simulink model "RIP"  (R2023b)
settings: Solver=ode23t  StartTime=0.0  StopTime=inf  RelTol=1e-3
model workspace: external: MATLAB File D:\AHMED\ASU\STUDENT\5. SENIOR 2\Semester 9\Hybrid Systems Control\Major Task\5. Simulink & GUI (V2)\Simulation\RIP_DataFile.m (data not in the file)
undefined symbols (not defined in the file or in its folder): k, smiData, X, Y, Z
libraries: sm_lib x16, nesl_utility x7, ee_lib x5, fl_lib x4, eeGeneralControl x2
settings Model: Creator=ahmed  LastModifiedBy=ahmed
settings ExplorerConfigSet: InternalSimMechanicsExplorerSettings="<ExplorerConfiguration><canonicalview>planar_xy</canonicalview><AnimationSetting><BasePlaybackSpeed>1.0</BasePlaybackSpeed><PlaybackSpeedFactor>1.0</PlaybackSpeedFactor></AnimationSetting><TilePanel><TileInfo><Tiles Columns=\"1\" Count=\"1\" Rows=\"1\"><Column Weight=\"1\"/><Row Weight=\"1\"/><Tile Height=\"1\" Width=\"1\" X=\"0\" Y=\"0\"/></Tiles></TileInfo><SceneInfo><SceneViewer><BGColor><R>0.60000002384185791</R><G>0.60000002384185791</G><B>0.60000002384185791</B></BGColor><Camera><DoPerspective>off</DoPerspective><Position><X>0.452835062728077831</X><Y>0.750380680384863274</Y><Z>0.622835063996346916</Z></Position><Center><X>-0.124515206461548039</X><Y>0.173030411195237543</Y><Z>0.0454847948067210878</Z></Center><Up><X>-0.408248290463863073</X><Y>0.816496580927726145</Y><Z>-0.408248290463863073</Z></Up><ViewLimDist>1</ViewLimDist><YLim>0.255279300212860105</YLim><XLim>0.46883025327554112</XLim></Camera></SceneViewer></SceneInfo></TilePanel><MechEditorPanel><Cameras/><GfxPanelCameraMap/><VideoCreator><PlaybackSpeedRatio>1.0</PlaybackSpeedRatio><FrameRate>30</FrameRate><VideoFormat>Motion JPEG AVI</VideoFormat><FrameSize>auto</FrameSize></VideoCreator></MechEditorPanel></ExplorerConfiguration>"

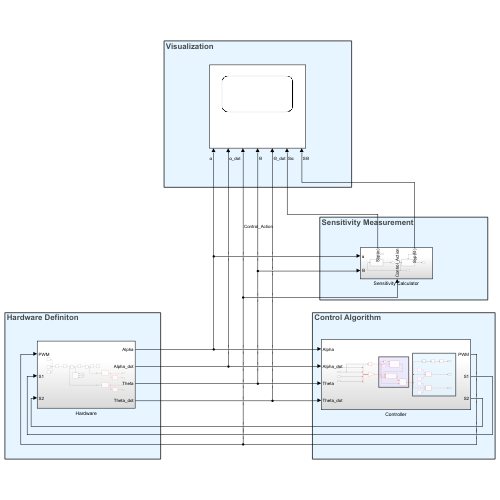
[thumbnail: Simulink's stored preview of the top-level diagram]
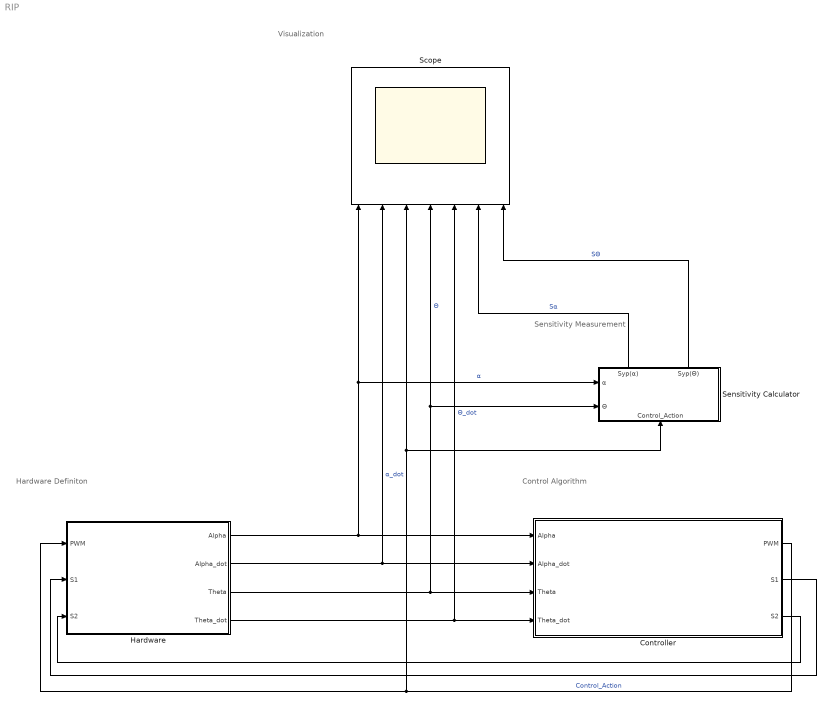
== system RIP ==
  note: Visualization
  note: Control Algorithm
  note: Hardware Definiton
  note: Sensitivity Measurement
  Controller : Subsystem
  Hardware : Subsystem
  Scope : Scope  NumInputPorts=7
  Sensitivity Calculator : Subsystem
      settings: PortSchema="{\"entries\":[{\"content\":{\"sides\":[{\"content\":{\"connectorIds\":[\"In1\",\"In2\"]},\"type\":\"ConnectorPlacement.EquallySpacedRectSide\",\"uuid\":\"a2b76d68-7d10-4964-b793-c2b104dfa3db\"},{\"content\":{\"side\":\"RIGHT\"},\"type\":\"ConnectorPlacement.EquallySpacedRectSide\",\"uuid\":\"40182234-6568-4180-b40e-3a35cefd8a8d\"},{\"content\":{\"connectorIds\":[\"Out1\",\"Out2\"],\"side\":\"TOP\"},\"type\":\"ConnectorPlacement.EquallySpacedRectSide\",\"uuid\":\"a20c4198-3069-423f-ae66-29ef70cd25fc\"},{\"content\":{\"connectorIds\":[\"In3\"],\"side\":\"BOTTOM\"},\"type\":\"ConnectorPlacement.EquallySpacedRectSide\",\"uuid\":\"777a26e0-898e-40e7-afe2-be20485a2fc9\"}]},\"type\":\"ConnectorPlacement.EquallySpacedConnector\",\"uuid\":\"2eeb0501-ac65-4270-abcc-9f050e1f1400\"}],\"packageUris\":[\"http://schema.mathworks.com/mf0/Connector/R2020b\"],\"version\":\"1.0\"}"
  wires:
  Hardware/1(Alpha) -> Controller/1(Alpha), Scope/1, Sensitivity Calculator/1(α)  "α"
  Hardware/2(Alpha_dot) -> Controller/2(Alpha_dot), Scope/2  "α_dot"
  Hardware/3(Theta) -> Controller/3(Theta), Sensitivity Calculator/2(Θ), Scope/4  "Θ"
  Hardware/4(Theta_dot) -> Controller/4(Theta_dot), Scope/5  "Θ_dot"
  Controller/1(PWM) -> Scope/3, Sensitivity Calculator/3(Control_Action), Hardware/1(PWM)  "Control_Action"
  Controller/2(S1) -> Hardware/2(S1)
  Controller/3(S2) -> Hardware/3(S2)
  Sensitivity Calculator/1(Syp(α)) -> Scope/6  "Sα"
  Sensitivity Calculator/2(Syp(Θ)) -> Scope/7  "SΘ"

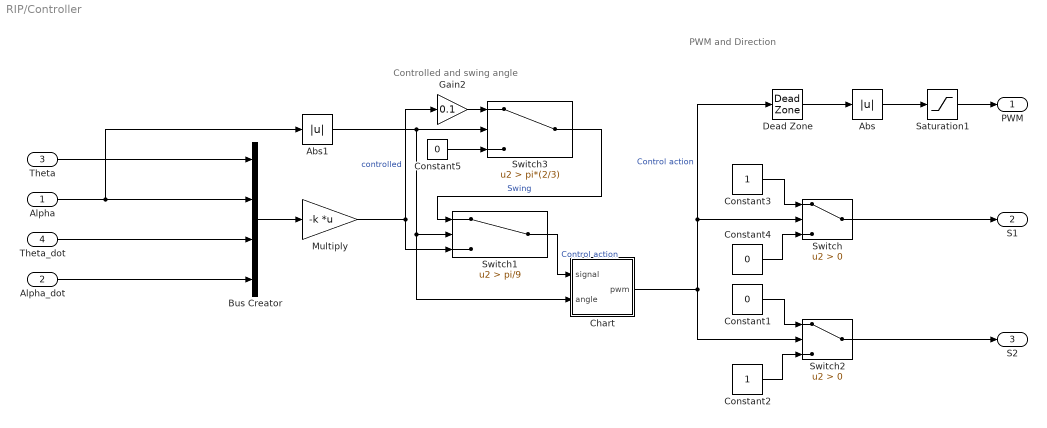
== system RIP/Controller ==
  note: Controlled and swing angle
  note: PWM and Direction
  Alpha : Inport
  Alpha_dot : Inport  Port=2
  Theta : Inport  Port=3
  Theta_dot : Inport  Port=4
  Abs : Abs  OutDataTypeStr=double  SaturateOnIntegerOverflow=off
  Abs1 : Abs  OutDataTypeStr=double  SaturateOnIntegerOverflow=off
  Bus Creator : BusCreator  Inputs=4
  Chart : Stateflow chart  TreatAsAtomicUnit=on  SystemSampleTime=0.001
      settings: PortSchema="{\"entries\":[{\"content\":{\"sides\":[{\"content\":{\"connectorIds\":[\"In2\",\"In1\"]},\"type\":\"ConnectorPlacement.EquallySpacedRectSide\",\"uuid\":\"28e2c2a8-bb0f-48a1-9e94-8475c8c1f5fa\"},{\"content\":{\"connectorIds\":[\"Out1\"],\"side\":\"RIGHT\"},\"type\":\"ConnectorPlacement.EquallySpacedRectSide\",\"uuid\":\"685929b8-ebaf-43fb-a3f1-f9f50dd919ab\"},{\"content\":{\"side\":\"TOP\"},\"type\":\"ConnectorPlacement.EquallySpacedRectSide\",\"uuid\":\"2e9fc888-3b47-4e34-86c2-38ebf694bde1\"}]},\"type\":\"ConnectorPlacement.EquallySpacedConnector\",\"uuid\":\"7dd89bc6-9eab-4521-81b3-1baa801bda82\"}],\"packageUris\":[\"http://schema.mathworks.com/mf0/Connector/R2020b\"],\"version\":\"1.0\"}"
  Constant1 : Constant  Value=0
  Constant2 : Constant
  Constant3 : Constant
  Constant4 : Constant  Value=0
  Constant5 : Constant  Value=0
  Dead Zone : DeadZone  LowerValue=-0  UpperValue=0
  Gain2 : Gain  Gain=0.1  OutDataTypeStr=double
  Multiply : Gain  Gain=-k  Multiplication=Matrix(K*u) (u vector)  OutDataTypeStr=double
  Saturation1 : Saturate  UpperLimit=255  LowerLimit=0
  Switch : Switch  Criteria=u2 > Threshold  OutDataTypeStr=double  SaturateOnIntegerOverflow=off  InputSameDT=off
  Switch1 : Switch  Criteria=u2 > Threshold  Threshold=pi/9  OutDataTypeStr=double  SaturateOnIntegerOverflow=off  InputSameDT=off
  Switch2 : Switch  Criteria=u2 > Threshold  OutDataTypeStr=double  SaturateOnIntegerOverflow=off  InputSameDT=off
  Switch3 : Switch  Criteria=u2 > Threshold  Threshold=pi*(2/3)  OutDataTypeStr=double  SaturateOnIntegerOverflow=off  InputSameDT=off
  PWM : Outport
  S1 : Outport  Port=2
  S2 : Outport  Port=3
  wires:
  Switch3/1 -> Switch1/1  "Swing"
  Bus Creator/1 -> Multiply/1
  Constant5/1 -> Switch3/3
  Abs1/1 -> Chart/1(angle), Switch1/2, Switch3/2
  Switch1/1 -> Chart/2(signal)  "Control action"
  Abs/1 -> Saturation1/1
  Constant4/1 -> Switch/3
  Multiply/1 -> Switch1/3, Gain2/1  "controlled"
  Chart/1(pwm) -> Switch2/2, Dead Zone/1, Switch/2  "Control action"
  Constant3/1 -> Switch/1
  Gain2/1 -> Switch3/1
  Theta_dot/1 -> Bus Creator/3
  Alpha/1 -> Abs1/1, Bus Creator/2
  Alpha_dot/1 -> Bus Creator/4
  Theta/1 -> Bus Creator/1
  Constant2/1 -> Switch2/3
  Constant1/1 -> Switch2/1
  Switch/1 -> S1/1
  Switch2/1 -> S2/1
  Saturation1/1 -> PWM/1
  Dead Zone/1 -> Abs/1

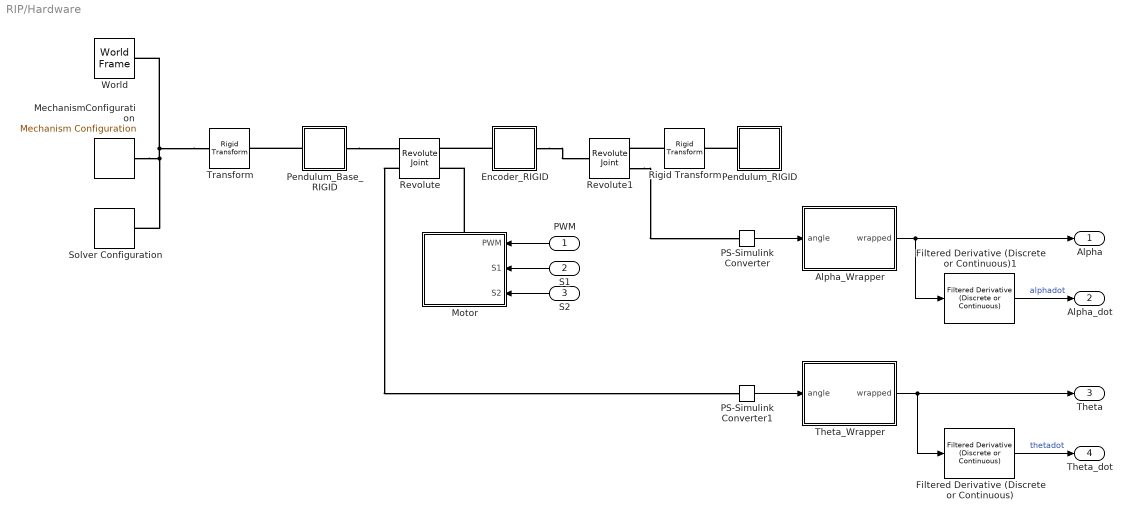
== system RIP/Hardware ==
  PWM : Inport
  S1 : Inport  Port=2
  S2 : Inport  Port=3
  Alpha_Wrapper : Subsystem
  Encoder_RIGID : Subsystem
  Filtered Derivative (Discrete or Continuous) : eeGeneralControl/Filtered Derivative (Discrete or Continuous)  K=1  T=0.01  B=inf  A=-inf  minRatio=10  init_option=Inherited from block input  x0=0  Ts=0.001
  Filtered Derivative (Discrete or Continuous)1 : eeGeneralControl/Filtered Derivative (Discrete or Continuous)  K=1  T=0.01  B=inf  A=-inf  minRatio=10  init_option=Inherited from block input  x0=0  Ts=0.001
  MechanismConfiguration : sm_lib/Utilities/Mechanism Configuration  UniformGravity=Constant  GravityVector=[0 -9.80665 0]  GravityVectorUnits=m/s^2  LinearizationDelta=0.001  JointModeTransitionNonlinearIterations=2
  Motor : Subsystem
      settings: PortSchema="{\"entries\":[{\"content\":{\"sides\":[{\"content\":{\"connectorIds\":[\"In1\",\"In2\",\"In3\"]},\"type\":\"ConnectorPlacement.EquallySpacedRectSide\",\"uuid\":\"136519c0-e6e7-4f60-8118-7da421ad854f\"},{\"content\":{\"side\":\"RIGHT\"},\"type\":\"ConnectorPlacement.EquallySpacedRectSide\",\"uuid\":\"84029570-417a-4f29-8386-7a87dba75fb0\"},{\"content\":{\"connectorIds\":[\"LConn1\"],\"side\":\"TOP\"},\"type\":\"ConnectorPlacement.EquallySpacedRectSide\",\"uuid\":\"71041409-d84d-47e2-8404-9c3758d614df\"},{\"content\":{\"side\":\"BOTTOM\"},\"type\":\"ConnectorPlacement.EquallySpacedRectSide\",\"uuid\":\"d454fdba-e8a0-47dc-974f-85f7355ee0b2\"}]},\"type\":\"ConnectorPlacement.EquallySpacedConnector\",\"uuid\":\"ea5fe486-c99a-4ca4-a0d9-4b6f02af3ced\"}],\"packageUris\":[\"http://schema.mathworks.com/mf0/Connector/R2020b\"],\"version\":\"1.0\"}"
  PS-Simulink Converter : nesl_utility/PS-Simulink Converter  PhysicalDomain=network_engine_domain  SubClassName=ps_output  LeftPortType=input  RightPortType=output  PseudoPeriodic=off  Frequencies=[]  VectorFormat=inherit  Unit=inherit  AffineConversion=off
  PS-Simulink Converter1 : nesl_utility/PS-Simulink Converter  PhysicalDomain=network_engine_domain  SubClassName=ps_output  LeftPortType=input  RightPortType=output  PseudoPeriodic=off  Frequencies=[]  VectorFormat=inherit  Unit=inherit  AffineConversion=off
  Pendulum_Base_RIGID : Subsystem
  Pendulum_RIGID : Subsystem
  Revolute : sm_lib/Joints/Revolute Joint  JointMode=Normal  SenseConstraintForce=off  SenseConstraintForceX=off  SenseConstraintForceY=off  SenseConstraintForceZ=off  SenseConstraintTorque=off  SenseConstraintTorqueX=off  SenseConstraintTorqueY=off  SenseConstraintTorqueZ=off  SenseTotalForce=off  SenseTotalForceX=off  SenseTotalForceY=off  SenseTotalForceZ=off  SenseTotalTorque=off  SenseTotalTorqueX=off  SenseTotalTorqueY=off  SenseTotalTorqueZ=off  CompositeWrenchDir=FollowerOnBase  CompositeWrenchFrame=BaseFrame  EquilibriumPosition=0  EquilibriumPositionUnits=deg  SpringStiffness=0  SpringStiffnessUnits=N*m/deg  DampingCoefficient=0  DampingCoefficientUnits=N*m/(deg/s)  TorqueActuationMode=InputTorque  MotionActuationMode=ComputedMotion  SensePosition=on  SenseVelocity=off  SenseAcceleration=off  SenseTorqueForce=off  SenseLowerLimitTorqueForce=off  SenseUpperLimitTorqueForce=off  LowerLimitSpecify=off  LowerLimitBound=-90  LowerLimitBoundUnits=deg  LowerLimitStiffness=1e4  LowerLimitStiffnessUnits=N*m/deg  LowerLimitDamping=10  LowerLimitDampingUnits=N*m/(deg/s)  LowerLimitTransitionRegionWidth=0.1  LowerLimitTransitionRegionWidthUnits=deg  UpperLimitSpecify=off  UpperLimitBound=90  UpperLimitBoundUnits=deg  UpperLimitStiffness=1e4  UpperLimitStiffnessUnits=N*m/deg  UpperLimitDamping=10  UpperLimitDampingUnits=N*m/(deg/s)  UpperLimitTransitionRegionWidth=0.1  UpperLimitTransitionRegionWidthUnits=deg  PositionTargetSpecify=on  PositionTargetPriority=Low  PositionTargetValue=smiData.RevoluteJoint(1).Rz.Pos  PositionTargetValueUnits=deg  VelocityTargetSpecify=off  VelocityTargetPriority=High  VelocityTargetValue=0  VelocityTargetValueUnits=deg/s
  Revolute1 : sm_lib/Joints/Revolute Joint  JointMode=Normal  SenseConstraintForce=off  SenseConstraintForceX=off  SenseConstraintForceY=off  SenseConstraintForceZ=off  SenseConstraintTorque=off  SenseConstraintTorqueX=off  SenseConstraintTorqueY=off  SenseConstraintTorqueZ=off  SenseTotalForce=off  SenseTotalForceX=off  SenseTotalForceY=off  SenseTotalForceZ=off  SenseTotalTorque=off  SenseTotalTorqueX=off  SenseTotalTorqueY=off  SenseTotalTorqueZ=off  CompositeWrenchDir=FollowerOnBase  CompositeWrenchFrame=BaseFrame  EquilibriumPosition=0  EquilibriumPositionUnits=deg  SpringStiffness=0  SpringStiffnessUnits=N*m/deg  DampingCoefficient=0  DampingCoefficientUnits=N*m/(deg/s)  TorqueActuationMode=NoTorque  MotionActuationMode=ComputedMotion  SensePosition=on  SenseVelocity=off  SenseAcceleration=off  SenseTorqueForce=off  SenseLowerLimitTorqueForce=off  SenseUpperLimitTorqueForce=off  LowerLimitSpecify=off  LowerLimitBound=-90  LowerLimitBoundUnits=deg  LowerLimitStiffness=1e4  LowerLimitStiffnessUnits=N*m/deg  LowerLimitDamping=10  LowerLimitDampingUnits=N*m/(deg/s)  LowerLimitTransitionRegionWidth=0.1  LowerLimitTransitionRegionWidthUnits=deg  UpperLimitSpecify=off  UpperLimitBound=90  UpperLimitBoundUnits=deg  UpperLimitStiffness=1e4  UpperLimitStiffnessUnits=N*m/deg  UpperLimitDamping=10  UpperLimitDampingUnits=N*m/(deg/s)  UpperLimitTransitionRegionWidth=0.1  UpperLimitTransitionRegionWidthUnits=deg  PositionTargetSpecify=on  PositionTargetPriority=Low  PositionTargetValue=smiData.RevoluteJoint(2).Rz.Pos  PositionTargetValueUnits=deg  VelocityTargetSpecify=off  VelocityTargetPriority=High  VelocityTargetValue=0  VelocityTargetValueUnits=deg/s
  Rigid Transform : sm_lib/Frames and Transforms/Rigid Transform  TranslationMethod=None  TranslationStandardOffset=0  TranslationStandardOffsetUnits=m  TranslationStandardAxis=+Z  TranslationCartesianOffset=[0 0 0]  TranslationCartesianOffsetUnits=m  TranslationROffset=0  TranslationROffsetUnits=m  TranslationZOffset=0  TranslationZOffsetUnits=m  TranslationThetaOffset=0  TranslationThetaOffsetUnits=deg  RotationMethod=StandardAxis  RotationAngleUnits=deg  RotationStandardAxis=+Z  RotationAngle=0  RotationArbitraryAxis=[0 0 1]  FollAlignAxisA=+X  BaseAlignAxisA=+Y  FollAlignAxisB=+Y  BaseAlignAxisB=+Z  RotationSequenceAxes=FollowerAxes  RotationSequence=XYX  RotationSequenceAngles=[0 0 0]  RotationSequenceAnglesUnits=deg  RotationMatrix=[1 0 0; 0 1 0; 0 0 1]  Quaternion=[1 0 0 0]
  Solver Configuration : nesl_utility/Solver Configuration  PhysicalDomain=network_engine_domain  SubClassName=solver  LeftPortType=input  RightPortType=generic  Tones=[]  Harmonics=[]  SimulateNoise=off  Profile=off  UseLocalSampling=off  EnableSwitchedLinearOptims=on  FrequencyDomain=off  UseCCode=off  RelTol=0.001  AbsTol=0.001  MinStep=1e-09  ToWorkspace=off  RevertToSquareIcSolve=off  NumHomotopyIterations=100  PhasorMode=off  PhasorModeNumHarmonics=1  ConsistencySolver=NEWTON_XTOL_AFTER_FTOL  IndexReductionMethod=DerivativeReplacement  DoDC=off  ResidualTolerance=1e-09  ConsistencyTolSource=GLOBAL  ConsistencyAbsTol=0.001  ConsistencyRelTol=0.001  ConsistencyTolFactor=0.001  UseLocalSolver=off  LocalSolverChoice=NE_BACKWARD_EULER_ADVANCER  ResolveIndetEquations=on  FunctionEvalNumThread=1  LocalSolverSampleTime=0.001  DoFixedCost=off  MaxNonlinIter=3  MaxModeIter=2  ComputeImpulses=off  ImpulseIterations=2  LinearAlgebra=auto  LinearAlgebraNumThread=0  EquationFormulation=NE_TIME_EF  DelaysMemoryBudget=1024  AutomaticFiltering=on  FilteringTimeConstant=0.001  PartitionStorageMethod=AS_NEEDED  PartitionMemoryBudget=1024  PartitionMethod=ROBUST  MultibodyUseLocalSolver=off  MultibodyLocalSolverChoice=ODE1  MultibodyLocalSolverSampleTime=0.001
  Theta_Wrapper : Subsystem
  Transform : sm_lib/Frames and Transforms/Rigid Transform  TranslationMethod=Cartesian  TranslationStandardOffset=0  TranslationStandardOffsetUnits=m  TranslationStandardAxis=+Z  TranslationCartesianOffset=smiData.RigidTransform(5).translation  TranslationCartesianOffsetUnits=mm  TranslationROffset=0  TranslationROffsetUnits=m  TranslationZOffset=0  TranslationZOffsetUnits=m  TranslationThetaOffset=0  TranslationThetaOffsetUnits=deg  RotationMethod=ArbitraryAxis  RotationAngleUnits=rad  RotationStandardAxis=+Z  RotationAngle=smiData.RigidTransform(5).angle  RotationArbitraryAxis=smiData.RigidTransform(5).axis  FollAlignAxisA=+X  BaseAlignAxisA=+Y  FollAlignAxisB=+Y  BaseAlignAxisB=+Z  RotationSequenceAxes=FollowerAxes  RotationSequence=XYX  RotationSequenceAngles=[0 0 0]  RotationSequenceAnglesUnits=deg  RotationMatrix=[1 0 0; 0 1 0; 0 0 1]  Quaternion=[1 0 0 0]
  World : sm_lib/Frames and Transforms/World Frame
  Alpha : Outport
  Alpha_dot : Outport  Port=2
  Theta : Outport  Port=3
  Theta_dot : Outport  Port=4
  wires:
  PS-Simulink Converter/1 -> Alpha_Wrapper/1(angle)
  Alpha_Wrapper/1(wrapped) -> Filtered Derivative (Discrete or Continuous)1/1, Alpha/1
  PS-Simulink Converter1/1 -> Theta_Wrapper/1(angle)
  Theta_Wrapper/1(wrapped) -> Filtered Derivative (Discrete or Continuous)/1, Theta/1
  Filtered Derivative (Discrete or Continuous)1/1 -> Alpha_dot/1  "alphadot"
  Filtered Derivative (Discrete or Continuous)/1 -> Theta_dot/1  "thetadot"
  PWM/1 -> Motor/1(PWM)
  S1/1 -> Motor/2(S1)
  S2/1 -> Motor/3(S2)
  connections:
  Pendulum_Base_RIGID/LConn1 -- Transform/RConn1
  Transform/LConn1 -- MechanismConfiguration/RConn1 -- Solver Configuration/RConn1 -- World/RConn1
  Pendulum_RIGID/LConn1 -- Rigid Transform/RConn1
  Encoder_RIGID/LConn1 -- Revolute/LConn1
  Encoder_RIGID/RConn1 -- Revolute1/LConn1
  Pendulum_Base_RIGID/RConn1 -- Revolute/RConn1
  Motor/LConn1 -- Revolute/LConn2
  Revolute1/RConn2 -- PS-Simulink Converter/LConn1
  Revolute/RConn2 -- PS-Simulink Converter1/LConn1
  Rigid Transform/LConn1 -- Revolute1/RConn1

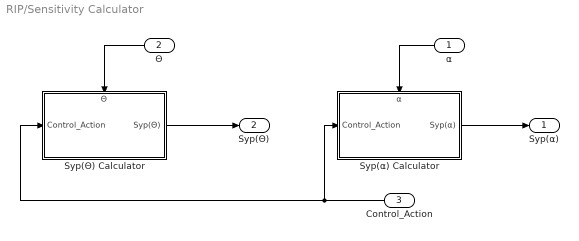
== system RIP/Sensitivity Calculator ==
  α : Inport
  Θ : Inport  Port=2
  Control_Action : Inport  Port=3
  Syp(Θ) Calculator : Subsystem
      settings: PortSchema="{\"entries\":[{\"content\":{\"sides\":[{\"content\":{\"connectorIds\":[\"In1\"]},\"type\":\"ConnectorPlacement.EquallySpacedRectSide\",\"uuid\":\"27eef1b6-850a-46d6-9e95-ce758ac832b8\"},{\"content\":{\"connectorIds\":[\"Out1\"],\"side\":\"RIGHT\"},\"type\":\"ConnectorPlacement.EquallySpacedRectSide\",\"uuid\":\"734eba0d-f9a1-4135-9d68-f935bde65952\"},{\"content\":{\"connectorIds\":[\"In2\"],\"side\":\"TOP\"},\"type\":\"ConnectorPlacement.EquallySpacedRectSide\",\"uuid\":\"fed29cd1-b455-4536-ac07-b773a13de225\"},{\"content\":{\"side\":\"BOTTOM\"},\"type\":\"ConnectorPlacement.EquallySpacedRectSide\",\"uuid\":\"ff06e8fe-5214-4c91-89f5-2483b4ea0e77\"}]},\"type\":\"ConnectorPlacement.EquallySpacedConnector\",\"uuid\":\"8d69ee49-9479-43f0-b140-6ef95f82c74f\"}],\"packageUris\":[\"http://schema.mathworks.com/mf0/Connector/R2020b\"],\"version\":\"1.0\"}"
  Syp(α) Calculator : Subsystem
      settings: PortSchema="{\"entries\":[{\"content\":{\"sides\":[{\"content\":{\"connectorIds\":[\"In1\"]},\"type\":\"ConnectorPlacement.EquallySpacedRectSide\",\"uuid\":\"27eef1b6-850a-46d6-9e95-ce758ac832b8\"},{\"content\":{\"connectorIds\":[\"Out1\"],\"side\":\"RIGHT\"},\"type\":\"ConnectorPlacement.EquallySpacedRectSide\",\"uuid\":\"734eba0d-f9a1-4135-9d68-f935bde65952\"},{\"content\":{\"connectorIds\":[\"In2\"],\"side\":\"TOP\"},\"type\":\"ConnectorPlacement.EquallySpacedRectSide\",\"uuid\":\"fed29cd1-b455-4536-ac07-b773a13de225\"},{\"content\":{\"side\":\"BOTTOM\"},\"type\":\"ConnectorPlacement.EquallySpacedRectSide\",\"uuid\":\"ff06e8fe-5214-4c91-89f5-2483b4ea0e77\"}]},\"type\":\"ConnectorPlacement.EquallySpacedConnector\",\"uuid\":\"8d69ee49-9479-43f0-b140-6ef95f82c74f\"}],\"packageUris\":[\"http://schema.mathworks.com/mf0/Connector/R2020b\"],\"version\":\"1.0\"}"
  Syp(α) : Outport
  Syp(Θ) : Outport  Port=2
  wires:
  α/1 -> Syp(α) Calculator/2(α)
  Control_Action/1 -> Syp(Θ) Calculator/1(Control_Action), Syp(α) Calculator/1(Control_Action)
  Syp(Θ) Calculator/1(Syp(Θ)) -> Syp(Θ)/1
  Syp(α) Calculator/1(Syp(α)) -> Syp(α)/1
  Θ/1 -> Syp(Θ) Calculator/2(Θ)

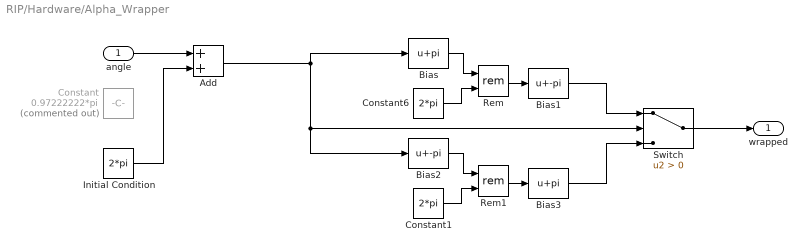
== system RIP/Hardware/Alpha_Wrapper ==
  angle : Inport
  Add : Sum
  Bias : Bias  Bias=pi  SaturateOnIntegerOverflow=off
  Bias1 : Bias  Bias=-pi  SaturateOnIntegerOverflow=off
  Bias2 : Bias  Bias=-pi  SaturateOnIntegerOverflow=off
  Bias3 : Bias  Bias=pi  SaturateOnIntegerOverflow=off
  Constant : Constant  Commented=on  Value=0.97222222*pi
  Constant1 : Constant  Value=2*pi
  Constant6 : Constant  Value=2*pi
  Initial Condition : Constant  Value=2*pi
  Rem : Math  Operator=rem  SignedPower=on
  Rem1 : Math  Operator=rem  SignedPower=on
  Switch : Switch  Criteria=u2 > Threshold  OutDataTypeStr=double  SaturateOnIntegerOverflow=off  InputSameDT=off
  wrapped : Outport
  wires:
  Constant6/1 -> Rem/2
  Bias1/1 -> Switch/1
  Bias/1 -> Rem/1
  Rem/1 -> Bias1/1
  Bias3/1 -> Switch/3
  Rem1/1 -> Bias3/1
  angle/1 -> Add/1
  Constant1/1 -> Rem1/2
  Bias2/1 -> Rem1/1
  Switch/1 -> wrapped/1
  Add/1 -> Bias2/1, Switch/2, Bias/1
  Initial Condition/1 -> Add/2

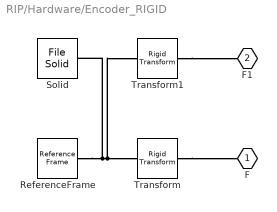
== system RIP/Hardware/Encoder_RIGID ==
  ReferenceFrame : sm_lib/Frames and Transforms/Reference Frame
  Solid : sm_lib/Body Elements/File Solid  ExtGeomFileName=Encoder_Default_sldprt.STEP  UnitType=FromFile  ExtGeomFileUnits=m  StepReaderType=HEX  ExportConvexHullGeometry=off  InertiaType=Custom  Mass=smiData.Solid(2).mass  MassUnits=kg  CenterOfMass=smiData.Solid(2).CoM  CenterOfMassUnits=mm  MomentsOfInertia=smiData.Solid(2).MoI  MomentsOfInertiaUnits=kg*mm^2  ProductsOfInertia=smiData.Solid(2).PoI  ProductsOfInertiaUnits=kg*mm^2  BasedOnType=DensityFromFile  Density=1000  DensityUnits=kg/m^3  DoExposeReferenceFrame=on  SerializedFrames=<Frames/>  GraphicType=FromGeometry  MarkerShape=Sphere  MarkerSize=10  GraphicVisPropType=SimpleVisualProperties  GraphicDiffuseColor=[0.0 0.4 0.8]  GraphicSpecularColor=[0.5 0.5 0.5 1.0]  GraphicAmbientColor=[0.15 0.15 0.15 1.0]  GraphicEmissiveColor=[0.0 0.0 0.0 1.0]  GraphicShininess=75  GraphicOpacity=smiData.Solid(2).opacity
  Transform : sm_lib/Frames and Transforms/Rigid Transform  TranslationMethod=Cartesian  TranslationStandardOffset=0  TranslationStandardOffsetUnits=m  TranslationStandardAxis=+Z  TranslationCartesianOffset=smiData.RigidTransform(1).translation  TranslationCartesianOffsetUnits=mm  TranslationROffset=0  TranslationROffsetUnits=m  TranslationZOffset=0  TranslationZOffsetUnits=m  TranslationThetaOffset=0  TranslationThetaOffsetUnits=deg  RotationMethod=ArbitraryAxis  RotationAngleUnits=rad  RotationStandardAxis=+Z  RotationAngle=smiData.RigidTransform(1).angle  RotationArbitraryAxis=smiData.RigidTransform(1).axis  FollAlignAxisA=+X  BaseAlignAxisA=+Y  FollAlignAxisB=+Y  BaseAlignAxisB=+Z  RotationSequenceAxes=FollowerAxes  RotationSequence=XYX  RotationSequenceAngles=[0 0 0]  RotationSequenceAnglesUnits=deg  RotationMatrix=[1 0 0; 0 1 0; 0 0 1]  Quaternion=[1 0 0 0]
  Transform1 : sm_lib/Frames and Transforms/Rigid Transform  TranslationMethod=Cartesian  TranslationStandardOffset=0  TranslationStandardOffsetUnits=m  TranslationStandardAxis=+Z  TranslationCartesianOffset=smiData.RigidTransform(3).translation  TranslationCartesianOffsetUnits=mm  TranslationROffset=0  TranslationROffsetUnits=m  TranslationZOffset=0  TranslationZOffsetUnits=m  TranslationThetaOffset=0  TranslationThetaOffsetUnits=deg  RotationMethod=ArbitraryAxis  RotationAngleUnits=rad  RotationStandardAxis=+Z  RotationAngle=smiData.RigidTransform(3).angle  RotationArbitraryAxis=smiData.RigidTransform(3).axis  FollAlignAxisA=+X  BaseAlignAxisA=+Y  FollAlignAxisB=+Y  BaseAlignAxisB=+Z  RotationSequenceAxes=FollowerAxes  RotationSequence=XYX  RotationSequenceAngles=[0 0 0]  RotationSequenceAnglesUnits=deg  RotationMatrix=[1 0 0; 0 1 0; 0 0 1]  Quaternion=[1 0 0 0]
  F : PMIOPort  Side=Left
  F1 : PMIOPort  Port=2  Side=Right
  connections:
  Solid/RConn1 -- ReferenceFrame/RConn1 -- Transform/LConn1 -- Transform1/LConn1
  Transform/RConn1 -- F/RConn1
  Transform1/RConn1 -- F1/RConn1

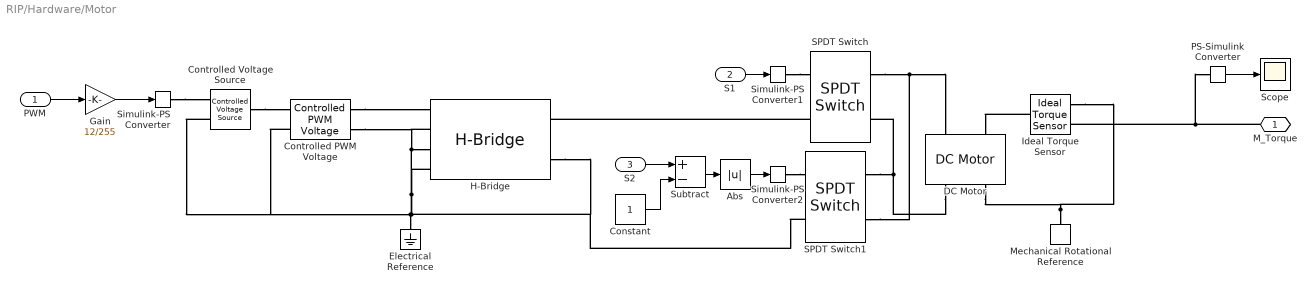
== system RIP/Hardware/Motor ==
  PWM : Inport
  S1 : Inport  Port=2
  S2 : Inport  Port=3
  Abs : Abs  SaturateOnIntegerOverflow=off
  Constant : Constant
  Controlled PWM Voltage : ee_lib/Integrated Circuits/Controlled PWM Voltage  F=1000 Hz  TD=0 s  pulse_width_offset=0 s  pulse_min=0 s  pwm_or_av=ee.enum.pwm_or_av.pwm  event_type=ee.enum.ic.event.asynchronous  sample_time=1e-6 s  Vmin=0 V  Vmax=12 V  Vm=12 V  u_min=0  u_max=1
  Controlled Voltage Source : fl_lib/Electrical/Electrical Sources/Controlled Voltage Source
  DC Motor : ee_lib/Electromechanical/Brushed Motors/DC Motor  field_option=ee.enum.field_option.pm  Rf=100 Ohm  Lf=1 H  Laf=0.15 H  If0=0 A  parameterization=ee.enum.dcparam_option.circuit_param  Ra=2 Ohm  La=0.23 H  emf_or_torque=ee.enum.emf_or_torque.ki  Kv=0.235 V/rpm  Ki=0.235 N*m/A  T_stall=0.24e-3 N*m  w_max=19100 rpm  w_rated=15000 rpm  P_rated=0.08 W  V_rated=1.5 V  lam_param=ee.enum.lam_param.damping  i_noload=0 A  V_i_noload=1.5 V  J=0.0052 kg*m^2  lam=0.01 N*m*s/rad  speed0=0 rpm  enable_fault_armature=simscape.enum.onoff.off  rev_faulted=1 / 3  G_faulted_armature=1e-5 S  fault_trigger_armature=ee.enum.faults.faultTrigger.temporal  t_fault_armature=1 s  max_permissible_current_armature=inf A  t_fail_on_current_armature=1 s  enable_fault_field=simscape.enum.onoff.off  G_faulted_field=1e-5 S  fault_trigger_field=ee.enum.faults.faultTrigger.temporal  t_fault_field=1 s  max_permissible_current_field=inf A  t_fail_on_current_field=1 s  fault_action=simscape.enum.assert.action.none  alpha=3.93e-3 1/K  Tmeas=25 degC  thermal_mass=100 J/K  initial_temperature=25 degC
  Electrical Reference : fl_lib/Electrical/Electrical Elements/Electrical Reference
  Gain : Gain  Gain=12/255
  H-Bridge : ee_lib/Semiconductors & Converters/Converters/H-Bridge  supply_ports=ee.enum.supply_ports.hidesupply  pwm_or_av=ee.enum.pwm_or_av.pwm  regenerative_braking_mode=ee.enum.converters.regenerative_braking_mode.depends_on_rev  discontinuous=ee.enum.current_profile.continuous  freewheeling_mode=ee.enum.converters.freewheeling_mode.one_switch_one_diode  Rload=10 Ohm  Lload=1e-5 H  F=10 kHz  Venable=0.001 V  Vmax=12 V  Vreverse=0.1 V  Vbrake=0.1 V  Vm=12 V  Ron=0.1 Ohm  Don=0.05 Ohm  Goff=1e-6 S  Tmeas=298.15 K  Ron2=0.1 Ohm  Don2=0.05 Ohm  Tmeas2=398.15 K  thermal_mass=100 J/K  initial_temperature=298.15 K
  Ideal Torque Sensor : fl_lib/Mechanical/Mechanical Sensors/Ideal Torque Sensor
  Mechanical Rotational Reference : fl_lib/Mechanical/Rotational Elements/Mechanical Rotational Reference
  PS-Simulink Converter : nesl_utility/PS-Simulink Converter  PhysicalDomain=network_engine_domain  SubClassName=ps_output  LeftPortType=input  RightPortType=output  PseudoPeriodic=off  Frequencies=[]  VectorFormat=inherit  Unit=inherit  AffineConversion=off
  SPDT Switch : ee_lib/Switches & Breakers/SPDT Switch  R_closed=0.01 Ohm  G_open=1e-6 S  Threshold=0.5 V  Width=0 V  model_dynamics=0  t_on=1e-3 s  t_off=1e-3 s  initial_vT=0 V
  SPDT Switch1 : ee_lib/Switches & Breakers/SPDT Switch  R_closed=0.01 Ohm  G_open=1e-6 S  Threshold=0.5 V  Width=0 V  model_dynamics=0  t_on=1e-3 s  t_off=1e-3 s  initial_vT=0 V
  Scope : Scope
  Simulink-PS Converter : nesl_utility/Simulink-PS Converter  PhysicalDomain=network_engine_domain  SubClassName=ps_input  LeftPortType=input  RightPortType=output  PseudoPeriodic=off  Frequencies=[]  NoiseDistribution=none  NoiseParameters=[]  Unit=1  AffineConversion=off  FilteringAndDerivatives=provide  SimscapeFilterOrder=1  InputFilterTimeConstant=0.001  UdotUserProvided=0
  Simulink-PS Converter1 : nesl_utility/Simulink-PS Converter  PhysicalDomain=network_engine_domain  SubClassName=ps_input  LeftPortType=input  RightPortType=output  PseudoPeriodic=off  Frequencies=[]  NoiseDistribution=none  NoiseParameters=[]  Unit=1  AffineConversion=off  FilteringAndDerivatives=provide  SimscapeFilterOrder=1  InputFilterTimeConstant=0.001  UdotUserProvided=0
  Simulink-PS Converter2 : nesl_utility/Simulink-PS Converter  PhysicalDomain=network_engine_domain  SubClassName=ps_input  LeftPortType=input  RightPortType=output  PseudoPeriodic=off  Frequencies=[]  NoiseDistribution=none  NoiseParameters=[]  Unit=1  AffineConversion=off  FilteringAndDerivatives=provide  SimscapeFilterOrder=1  InputFilterTimeConstant=0.001  UdotUserProvided=0
  Subtract : Sum  Inputs=+-
  M_Torque : PMIOPort  Side=Left
  wires:
  PWM/1 -> Gain/1
  Gain/1 -> Simulink-PS Converter/1
  S1/1 -> Simulink-PS Converter1/1
  S2/1 -> Subtract/1
  Constant/1 -> Subtract/2
  Subtract/1 -> Abs/1
  Abs/1 -> Simulink-PS Converter2/1
  PS-Simulink Converter/1 -> Scope/1
  connections:
  Electrical Reference/LConn1 -- Controlled PWM Voltage/LConn2 -- Controlled Voltage Source/RConn2 -- SPDT Switch1/LConn2 -- H-Bridge/RConn2 -- H-Bridge/LConn4 -- Controlled PWM Voltage/RConn2 -- H-Bridge/LConn2 -- H-Bridge/LConn3
  Mechanical Rotational Reference/LConn1 -- Ideal Torque Sensor/RConn1 -- DC Motor/RConn2
  Ideal Torque Sensor/LConn1 -- DC Motor/LConn2
  M_Torque/RConn1 -- PS-Simulink Converter/LConn1 -- Ideal Torque Sensor/RConn2
  Controlled PWM Voltage/RConn1 -- H-Bridge/LConn1
  Controlled Voltage Source/LConn1 -- Controlled PWM Voltage/LConn1
  Simulink-PS Converter/RConn1 -- Controlled Voltage Source/RConn1
  SPDT Switch/LConn2 -- H-Bridge/RConn1
  SPDT Switch/RConn1 -- DC Motor/LConn1 -- SPDT Switch1/RConn2
  DC Motor/RConn1 -- SPDT Switch/RConn2 -- SPDT Switch1/RConn1
  Simulink-PS Converter1/RConn1 -- SPDT Switch/LConn1
  Simulink-PS Converter2/RConn1 -- SPDT Switch1/LConn1

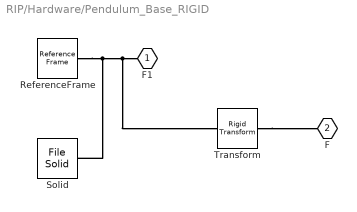
== system RIP/Hardware/Pendulum_Base_RIGID ==
  ReferenceFrame : sm_lib/Frames and Transforms/Reference Frame
  Solid : sm_lib/Body Elements/File Solid  ExtGeomFileName=P_Base_Default_sldprt.STEP  UnitType=FromFile  ExtGeomFileUnits=m  StepReaderType=HEX  ExportConvexHullGeometry=off  InertiaType=Custom  Mass=smiData.Solid(3).mass  MassUnits=kg  CenterOfMass=smiData.Solid(3).CoM  CenterOfMassUnits=mm  MomentsOfInertia=smiData.Solid(3).MoI  MomentsOfInertiaUnits=kg*mm^2  ProductsOfInertia=smiData.Solid(3).PoI  ProductsOfInertiaUnits=kg*mm^2  BasedOnType=DensityFromFile  Density=1000  DensityUnits=kg/m^3  DoExposeReferenceFrame=on  SerializedFrames=<Frames/>  GraphicType=FromGeometry  MarkerShape=Sphere  MarkerSize=10  GraphicVisPropType=SimpleVisualProperties  GraphicDiffuseColor=[0.0 0.2 0.2]  GraphicSpecularColor=[0.5 0.5 0.5 1.0]  GraphicAmbientColor=[0.15 0.15 0.15 1.0]  GraphicEmissiveColor=[0.0 0.0 0.0 1.0]  GraphicShininess=75  GraphicOpacity=smiData.Solid(3).opacity
  Transform : sm_lib/Frames and Transforms/Rigid Transform  TranslationMethod=Cartesian  TranslationStandardOffset=0  TranslationStandardOffsetUnits=m  TranslationStandardAxis=+Z  TranslationCartesianOffset=smiData.RigidTransform(2).translation  TranslationCartesianOffsetUnits=mm  TranslationROffset=0  TranslationROffsetUnits=m  TranslationZOffset=0  TranslationZOffsetUnits=m  TranslationThetaOffset=0  TranslationThetaOffsetUnits=deg  RotationMethod=ArbitraryAxis  RotationAngleUnits=rad  RotationStandardAxis=+Z  RotationAngle=smiData.RigidTransform(2).angle  RotationArbitraryAxis=smiData.RigidTransform(2).axis  FollAlignAxisA=+X  BaseAlignAxisA=+Y  FollAlignAxisB=+Y  BaseAlignAxisB=+Z  RotationSequenceAxes=FollowerAxes  RotationSequence=XYX  RotationSequenceAngles=[0 0 0]  RotationSequenceAnglesUnits=deg  RotationMatrix=[1 0 0; 0 1 0; 0 0 1]  Quaternion=[1 0 0 0]
  F1 : PMIOPort  Side=Left
  F : PMIOPort  Port=2  Side=Right
  connections:
  Solid/RConn1 -- ReferenceFrame/RConn1 -- Transform/LConn1 -- F1/RConn1
  Transform/RConn1 -- F/RConn1

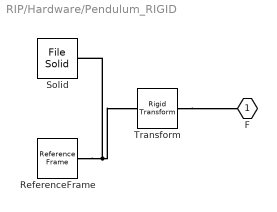
== system RIP/Hardware/Pendulum_RIGID ==
  ReferenceFrame : sm_lib/Frames and Transforms/Reference Frame
  Solid : sm_lib/Body Elements/File Solid  ExtGeomFileName=Pendulum_Default_sldprt.STEP  UnitType=FromFile  ExtGeomFileUnits=m  StepReaderType=HEX  ExportConvexHullGeometry=off  InertiaType=Custom  Mass=smiData.Solid(1).mass  MassUnits=kg  CenterOfMass=smiData.Solid(1).CoM  CenterOfMassUnits=mm  MomentsOfInertia=smiData.Solid(1).MoI  MomentsOfInertiaUnits=kg*mm^2  ProductsOfInertia=smiData.Solid(1).PoI  ProductsOfInertiaUnits=kg*mm^2  BasedOnType=DensityFromFile  Density=1000  DensityUnits=kg/m^3  DoExposeReferenceFrame=on  SerializedFrames=<Frames/>  GraphicType=FromGeometry  MarkerShape=Sphere  MarkerSize=10  GraphicVisPropType=SimpleVisualProperties  GraphicDiffuseColor=[0.8 0.8 0.8]  GraphicSpecularColor=[0.5 0.5 0.5 1.0]  GraphicAmbientColor=[0.15 0.15 0.15 1.0]  GraphicEmissiveColor=[0.0 0.0 0.0 1.0]  GraphicShininess=75  GraphicOpacity=smiData.Solid(1).opacity
  Transform : sm_lib/Frames and Transforms/Rigid Transform  TranslationMethod=Cartesian  TranslationStandardOffset=0  TranslationStandardOffsetUnits=m  TranslationStandardAxis=+Z  TranslationCartesianOffset=smiData.RigidTransform(4).translation  TranslationCartesianOffsetUnits=mm  TranslationROffset=0  TranslationROffsetUnits=m  TranslationZOffset=0  TranslationZOffsetUnits=m  TranslationThetaOffset=0  TranslationThetaOffsetUnits=deg  RotationMethod=ArbitraryAxis  RotationAngleUnits=rad  RotationStandardAxis=+Z  RotationAngle=smiData.RigidTransform(4).angle  RotationArbitraryAxis=smiData.RigidTransform(4).axis  FollAlignAxisA=+X  BaseAlignAxisA=+Y  FollAlignAxisB=+Y  BaseAlignAxisB=+Z  RotationSequenceAxes=FollowerAxes  RotationSequence=XYX  RotationSequenceAngles=[0 0 0]  RotationSequenceAnglesUnits=deg  RotationMatrix=[1 0 0; 0 1 0; 0 0 1]  Quaternion=[1 0 0 0]
  F : PMIOPort  Side=Left
  connections:
  Solid/RConn1 -- ReferenceFrame/RConn1 -- Transform/LConn1
  Transform/RConn1 -- F/RConn1

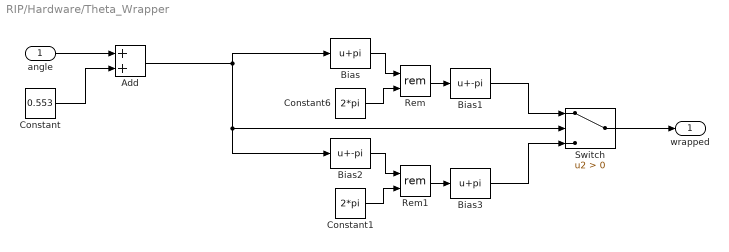
== system RIP/Hardware/Theta_Wrapper ==
  angle : Inport
  Add : Sum
  Bias : Bias  Bias=pi  SaturateOnIntegerOverflow=off
  Bias1 : Bias  Bias=-pi  SaturateOnIntegerOverflow=off
  Bias2 : Bias  Bias=-pi  SaturateOnIntegerOverflow=off
  Bias3 : Bias  Bias=pi  SaturateOnIntegerOverflow=off
  Constant : Constant  Value=0.553
  Constant1 : Constant  Value=2*pi
  Constant6 : Constant  Value=2*pi
  Rem : Math  Operator=rem  SignedPower=on
  Rem1 : Math  Operator=rem  SignedPower=on
  Switch : Switch  Criteria=u2 > Threshold  OutDataTypeStr=double  SaturateOnIntegerOverflow=off  InputSameDT=off
  wrapped : Outport
  wires:
  Constant6/1 -> Rem/2
  Bias1/1 -> Switch/1
  Bias/1 -> Rem/1
  Rem/1 -> Bias1/1
  Bias3/1 -> Switch/3
  Rem1/1 -> Bias3/1
  angle/1 -> Add/1
  Constant1/1 -> Rem1/2
  Bias2/1 -> Rem1/1
  Switch/1 -> wrapped/1
  Add/1 -> Bias2/1, Switch/2, Bias/1
  Constant/1 -> Add/2

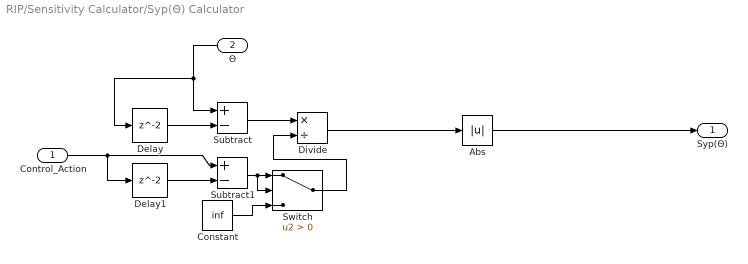
== system RIP/Sensitivity Calculator/Syp(Θ) Calculator ==
  Control_Action : Inport
  Θ : Inport  Port=2
  Abs : Abs  SaturateOnIntegerOverflow=off
  Constant : Constant  Value=inf
  Delay : Delay
  Delay1 : Delay
  Divide : Product  Inputs=*/
  Subtract : Sum  Inputs=+-
  Subtract1 : Sum  Inputs=+-
  Switch : Switch  Criteria=u2 > Threshold  SaturateOnIntegerOverflow=off  InputSameDT=off
  Syp(Θ) : Outport
  wires:
  Delay1/1 -> Subtract1/2
  Control_Action/1 -> Delay1/1, Subtract1/1
  Switch/1 -> Divide/2
  Subtract/1 -> Divide/1
  Θ/1 -> Subtract/1, Delay/1
  Constant/1 -> Switch/3
  Delay/1 -> Subtract/2
  Subtract1/1 -> Switch/2, Switch/1
  Divide/1 -> Abs/1
  Abs/1 -> Syp(Θ)/1

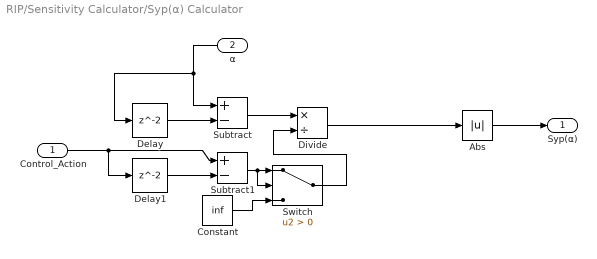
== system RIP/Sensitivity Calculator/Syp(α) Calculator ==
  Control_Action : Inport
  α : Inport  Port=2
  Abs : Abs  SaturateOnIntegerOverflow=off
  Constant : Constant  Value=inf
  Delay : Delay
  Delay1 : Delay
  Divide : Product  Inputs=*/
  Subtract : Sum  Inputs=+-
  Subtract1 : Sum  Inputs=+-
  Switch : Switch  Criteria=u2 > Threshold  SaturateOnIntegerOverflow=off  InputSameDT=off
  Syp(α) : Outport
  wires:
  Delay1/1 -> Subtract1/2
  Control_Action/1 -> Subtract1/1, Delay1/1
  Switch/1 -> Divide/2
  Subtract/1 -> Divide/1
  α/1 -> Subtract/1, Delay/1
  Constant/1 -> Switch/3
  Delay/1 -> Subtract/2
  Subtract1/1 -> Switch/2, Switch/1
  Divide/1 -> Abs/1
  Abs/1 -> Syp(α)/1

== stateflow chart RIP/Controller/Chart ==
  state Swing
    pwm=-150;
  state Stabilize
    pwm = signal
  (default) -> Swing
  Swing -> Stabilize : [angle < (pi)*(3/4)]
  Stabilize -> Swing : [[angle > (pi)*(3/4)] && after(3,sec)]
  data: pwm output; angle input; signal input
